simulink model "NadaDrive"  (R2020a)
settings: Solver=VariableStepAuto  StartTime=0.0  StopTime=inf  RelTol=1e-3
libraries: vrlib x1, sim3dlib x1, vdynlib x1, autolibshared x1
settings Model: Creator=Ivan  LastModifiedBy=Ivan

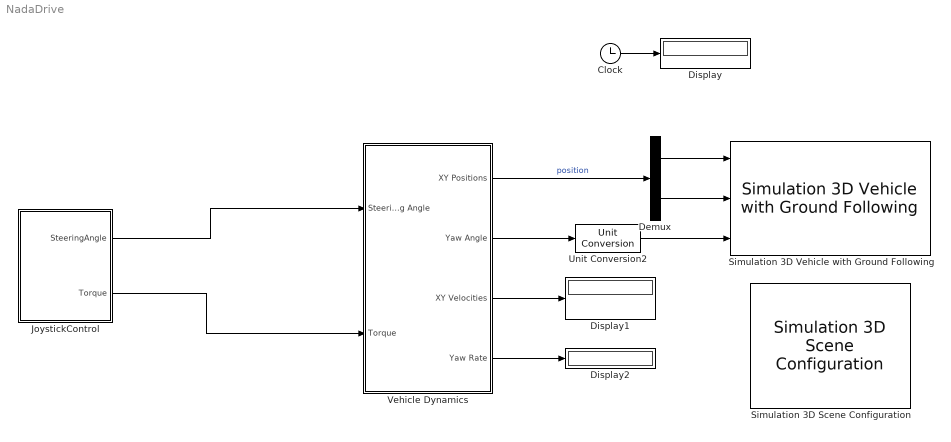
== system NadaDrive ==
  Clock : Clock
  Demux : Demux  Outputs=2
  Display : Display
  Display1 : Display
  Display2 : Display
  JoystickControl : Subsystem
  Simulation 3D Scene Configuration : sim3dlib/Simulation 3D Scene Configuration  Priority=0  ProjectFormat=Default Scenes  SceneDesc=Large parking lot  ProjectName=VehicleSimulation.exe  ScenePath=/Game/Maps/HwStrght  vehTagList={'Kia';'Scene Origin'}  vehTag=Kia  OpVisEn=off  Ts=1/100  EnableWindow=on  sensorTag=MainCamera1  sensorId=1  sensorName=MainCamera1  mountLoc=Origin  offsetFlag=off  tmountOffset=[0, 0, 0]  rmountOffset=[0, 0, 0]  HorizontalResolution=1280  VerticalResolution=720  HorizontalFOV=60  mountPoint=[0 0 0]  mountOrientation=[0 0 0]  aMode=2  ID=1
      settings: SourceProductBaseCode=DR,VE
  Simulation 3D Vehicle with Ground Following : vdynlib/Vehicle Scenarios/Sim3D/Sim3D Vehicle/Components/Simulation 3D Vehicle with Ground Following  Priority=-1  PassVehMesh=Muscle car  VehColor=Yellow  InitialPos=[0, 0, 0]  InitialRot=[0, 0, 0]  ActorName=Kia  SampleTime=-1  ActorType=SimulinkVehicle  ID=C  aMode=2  ActorTag=Kia  CoordinateScheme=SAE
      settings: SourceProductBaseCode=VE
  Unit Conversion2 : UnitConversion  OutputType=Inherit: Inherit via back propagation
  Vehicle Dynamics : Subsystem  VariantControl=VariantVDBS
  wires:
  JoystickControl/2(Torque) -> Vehicle Dynamics/2(Torque)
  Clock/1 -> Display/1
  Vehicle Dynamics/2(Yaw Angle) -> Unit Conversion2/1
  JoystickControl/1(SteeringAngle) -> Vehicle Dynamics/1(Steering Angle)
  Demux/1 -> Simulation 3D Vehicle with Ground Following/1
  Demux/2 -> Simulation 3D Vehicle with Ground Following/2
  Vehicle Dynamics/1(XY Positions) -> Demux/1  "position"
  Vehicle Dynamics/3(XY Velocities) -> Display1/1
  Vehicle Dynamics/4(Yaw Rate) -> Display2/1
  Unit Conversion2/1 -> Simulation 3D Vehicle with Ground Following/3

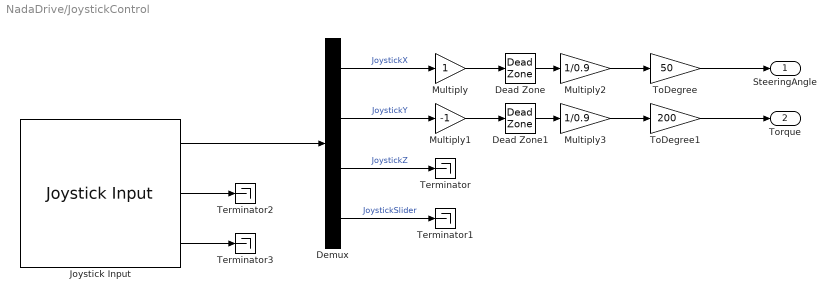
== system NadaDrive/JoystickControl ==
  Dead Zone : DeadZone  LowerValue=-0.1  UpperValue=0.1  SaturateOnIntegerOverflow=on
  Dead Zone1 : DeadZone  LowerValue=-0.1  UpperValue=0.1  SaturateOnIntegerOverflow=on
  Demux : Demux
  Joystick Input : vrlib/Joystick Input  joyid=1  adjustports=on  forcefeed=off
  Multiply : Gain
  Multiply1 : Gain  Gain=-1
  Multiply2 : Gain  Gain=1/0.9
  Multiply3 : Gain  Gain=1/0.9
  Terminator{,1..3} (4 alike) : Terminator
  ToDegree : Gain  Gain=50
  ToDegree1 : Gain  Gain=200
  SteeringAngle : Outport  Unit=deg
  Torque : Outport  Port=2  Unit=N*m
  wires:
  Multiply1/1 -> Dead Zone1/1
  Demux/2 -> Multiply1/1  "JoystickY"
  Demux/3 -> Terminator/1  "JoystickZ"
  Joystick Input/3 -> Terminator3/1
  Demux/4 -> Terminator1/1  "JoystickSlider"
  Demux/1 -> Multiply/1  "JoystickX"
  Joystick Input/2 -> Terminator2/1
  Multiply/1 -> Dead Zone/1
  Joystick Input/1 -> Demux/1
  Dead Zone/1 -> Multiply2/1
  Dead Zone1/1 -> Multiply3/1
  Multiply2/1 -> ToDegree/1
  Multiply3/1 -> ToDegree1/1
  ToDegree/1 -> SteeringAngle/1
  ToDegree1/1 -> Torque/1

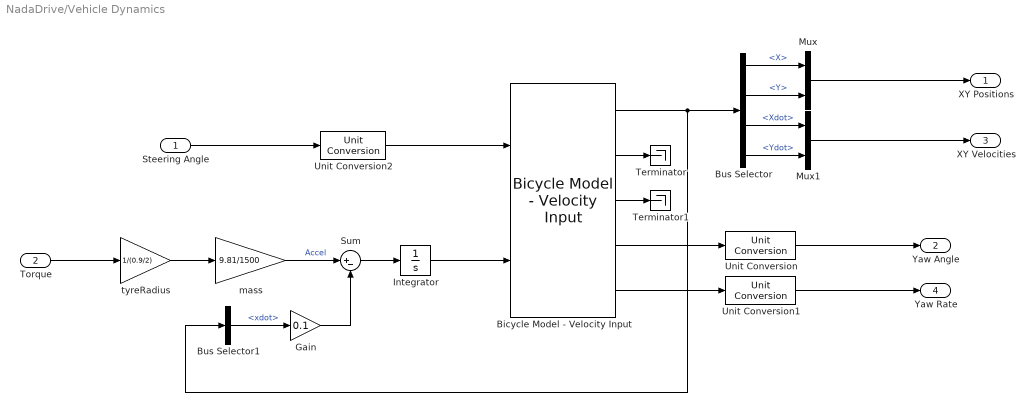
== system NadaDrive/Vehicle Dynamics ==
  Steering Angle : Inport  Unit=deg
  Torque : Inport  Port=2  Unit=N*m
  Bicycle Model - Velocity Input : autolibshared/Bicycle Model - Velocity Input  trackMode=Single (bicycle)  inputMode=External longitudinal forces  frontSteerMode=on  rearSteerMode=off  windMode=off  muMode=off  extFMode=off  extMMode=off  aMode=3  NF=2  NR=2  m=1500  a=1.2  b=1.6  h=0.35  X_o=0  xdot_o=0  CalphaMode=off  sigmaMode=on  w=[1.4,1.4]  Cy_f=19000  Cy_r=33000  sigma_f=.1  sigma_r=.1  alpha_f_brk=[-.1 .1]  Cy_f_data=[-9e3 9e3]  alpha_r_brk=[-.1 .1]  Cy_r_data=[-9e3 9e3]  Y_o=0  ydot_o=0  Izz=2875  psi_o=0*pi/180  r_o=0  Af=2  Cd=.3  Cl=.1  Cpm=.1  beta_w=[0:0.01:0.3]  Cs=[0:0.03:0.9]  Cym=[0:0.01:0.3]  Pabs=101325  Tair=273  g=9.81  mu=1  xdot_tol=.01  Fznom=5000  Fxtire_sat=1e6  Fytire_sat=1e6  longOff=0  latOff=0  vertOff=0
      settings: SourceProductBaseCode=PW,MT,VE,VP
  Bus Selector : BusSelector  OutputSignals=InertFrm.FrntAxl.Disp.X,InertFrm.FrntAxl.Disp.Y,InertFrm.FrntAxl.Vel.Xdot,InertFrm.FrntAxl.Vel.Ydot
  Bus Selector1 : BusSelector  OutputSignals=BdyFrm.Cg.Vel.xdot
  Gain : Gain  Gain=0.1
  Integrator : Integrator  LimitOutput=on  UpperSaturationLimit=100  LowerSaturationLimit=0
  Mux : Mux  Inputs=2
  Mux1 : Mux  Inputs=2
  Sum : Sum  Inputs=|+-
  Terminator : Terminator
  Terminator1 : Terminator
  Unit Conversion : UnitConversion  OutputType=Inherit: Inherit via back propagation
  Unit Conversion1 : UnitConversion  OutputType=Inherit: Inherit via back propagation
  Unit Conversion2 : UnitConversion  OutputType=Inherit: Inherit via back propagation
  mass : Gain  Gain=9.81/1500
  tyreRadius : Gain  Gain=1/(0.9/2)
  XY Positions : Outport  Unit=m  VectorParamsAs1DForOutWhenUnconnected=off
  Yaw Angle : Outport  Port=2  Unit=deg  VectorParamsAs1DForOutWhenUnconnected=off
  XY Velocities : Outport  Port=3  Unit=m/s  VectorParamsAs1DForOutWhenUnconnected=off
  Yaw Rate : Outport  Port=4  Unit=degree/s  VectorParamsAs1DForOutWhenUnconnected=off
  wires:
  Mux/1 -> XY Positions/1
  Mux1/1 -> XY Velocities/1
  Unit Conversion1/1 -> Yaw Rate/1
  Unit Conversion/1 -> Yaw Angle/1
  Bicycle Model - Velocity Input/2 -> Terminator/1
  Bicycle Model - Velocity Input/3 -> Terminator1/1
  Bicycle Model - Velocity Input/4 -> Unit Conversion/1
  Bicycle Model - Velocity Input/5 -> Unit Conversion1/1
  Bus Selector/1 -> Mux/1  "<X>"
  Bus Selector/2 -> Mux/2  "<Y>"
  Bus Selector/3 -> Mux1/1  "<Xdot>"
  Bus Selector/4 -> Mux1/2  "<Ydot>"
  Steering Angle/1 -> Unit Conversion2/1
  Integrator/1 -> Bicycle Model - Velocity Input/2
  Unit Conversion2/1 -> Bicycle Model - Velocity Input/1
  Bicycle Model - Velocity Input/1 -> Bus Selector1/1, Bus Selector/1
  Torque/1 -> tyreRadius/1
  Sum/1 -> Integrator/1
  Bus Selector1/1 -> Gain/1  "<xdot>"
  Gain/1 -> Sum/2
  mass/1 -> Sum/1  "Accel"
  tyreRadius/1 -> mass/1
